simulink model "simulation"  (R2015a)
settings: Solver=ode23tb  StartTime=0.0  StopTime=0.5  RelTol=1e-3
libraries: powerlib x16
settings Model: Creator=user  LastModifiedBy=user

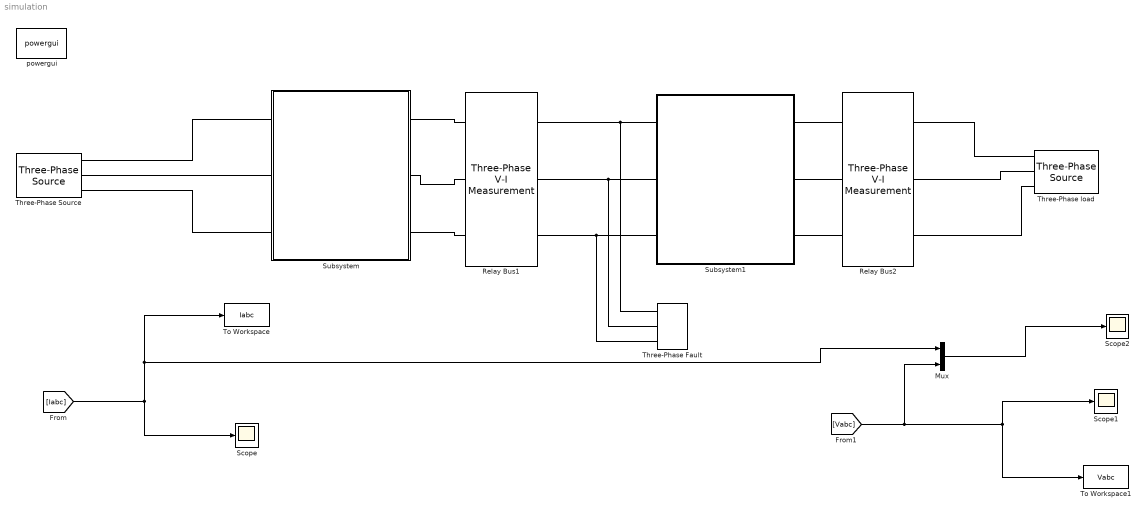
== system simulation ==
  Mux : Mux  Inputs=2
  Relay Bus1 : powerlib/Measurements/Three-Phase V-I Measurement  VoltageMeasurement=phase-to-phase  SetLabelV=on  LabelV=Vabc  Vpu=on  VpuLL=off  CurrentMeasurement=yes  SetLabelI=on  LabelI=Iabc  Ipu=on  Pbase=100e6  Vbase=500e3  OutputType=Complex  PhasorSimulation=off  PSBequivalent=0
  Relay Bus2 : powerlib/Measurements/Three-Phase V-I Measurement  VoltageMeasurement=no  SetLabelV=off  LabelV=Vabc  Vpu=on  VpuLL=off  CurrentMeasurement=no  SetLabelI=off  LabelI=Iabc  Ipu=on  Pbase=100e6  Vbase=500e3  OutputType=Complex  PhasorSimulation=off  PSBequivalent=0
  Scope : Scope
  Scope1 : Scope
  Scope2 : Scope
      settings: SaveName=ScopeData2
  Subsystem : Subsystem
  Subsystem1 : Subsystem
  Three-Phase Fault : powerlib/Elements/Three-Phase Fault  InitialStates=0  FaultA=on  FaultB=off  FaultC=off  GroundFault=on  SwitchTimes="[1/60  5/60]"  External=off  SwitchStatus=NaN  FaultResistance=0.001  GroundResistance=0.01  SnubberResistance=1e6  SnubberCapacitance=inf  Measurements=Fault voltages and currents
  Three-Phase Source : powerlib/Electrical Sources/Three-Phase Source  Voltage=500e3  PhaseAngle=0  Frequency=50  InternalConnection=Yg  SpecifyImpedance=off  Resistance=0.8929  Inductance=16.58e-3  ShortCircuitLevel=100e6  BaseVoltage=500e3  XRratio=7  BusType=swing  Pref=0  Qref=0  Qmin=-inf  Qmax=inf
  Three-Phase load : powerlib/Electrical Sources/Three-Phase Source  Voltage=500e3  PhaseAngle=-30  Frequency=50  InternalConnection=Yg  SpecifyImpedance=off  Resistance=0.8929  Inductance=16.58e-3  ShortCircuitLevel=100e6  BaseVoltage=500e3  XRratio=7  BusType=swing  Pref=0  Qref=0  Qmin=-inf  Qmax=inf
  To Workspace : ToWorkspace  VariableName=Iabc  SaveFormat=Timeseries
  To Workspace1 : ToWorkspace  VariableName=Vabc  SaveFormat=Timeseries
  powergui : powerlib/powergui  Priority=1  SimulationMode=Discrete  SolverType=Tustin/Backward Euler (TBE)  SampleTime=3e-5  frequency=60  SPID=off  DisableSnubberDevices=off  DisableRonSwitches=off  DisableVfSwitches=off  SwTol=0  DisplayEquations=off  Interpol=off  methode=off  Ts=100  FunctionMessages=off  echomessages=off  HookPort=off  EnableUseOfTLC=off  x0status=blocks  frequencyindice=50  Pbase=100e6  ErrMax=1e-4  Iterations=50  UnitsV=kV  UnitsW=MW  buscounter=0  RestoreLinks=warning  ResistiveCurrentMeasurement=off  Frange=[0:2:500]  Ylog=off  Xlog=on  ShowGrid=off  save=off  variable=ZData  structure=0  ZoomFFT=off  StartTime=0.0  cycles=1  DisplayStyle=1  fundamental=60  FreqAxis=off  MaxFrequency=1000  frequencyindicesteady=1  RmsSteady=1  display=off
  wires:
  [Iabc] -> Scope/1, Mux/1, To Workspace/1
  [Vabc] -> Mux/2, Scope1/1, To Workspace1/1
  Mux/1 -> Scope2/1
  connections:
  Relay Bus1/LConn2 -- Subsystem/RConn2
  Three-Phase Source/RConn1 -- Subsystem/LConn1
  Three-Phase Source/RConn2 -- Subsystem/LConn2
  Three-Phase Source/RConn3 -- Subsystem/LConn3
  Subsystem/RConn1 -- Relay Bus1/LConn1
  Subsystem/RConn3 -- Relay Bus1/LConn3
  Three-Phase load/RConn2 -- Relay Bus2/RConn2
  Three-Phase load/RConn3 -- Relay Bus2/RConn3
  Three-Phase load/RConn1 -- Relay Bus2/RConn1
  Subsystem1/RConn1 -- Relay Bus2/LConn1
  Subsystem1/RConn2 -- Relay Bus2/LConn2
  Subsystem1/RConn3 -- Relay Bus2/LConn3
  Relay Bus1/RConn2 -- Three-Phase Fault/LConn2 -- Subsystem1/LConn2
  Relay Bus1/RConn1 -- Three-Phase Fault/LConn1 -- Subsystem1/LConn1
  Relay Bus1/RConn3 -- Three-Phase Fault/LConn3 -- Subsystem1/LConn3

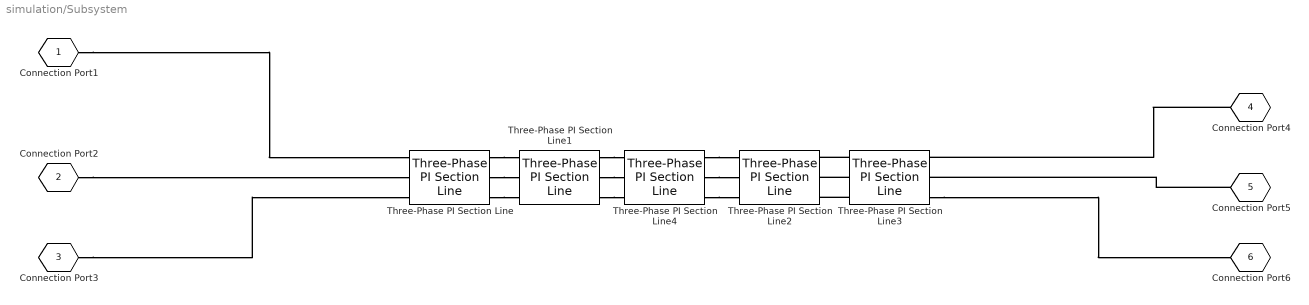
== system simulation/Subsystem ==
  Three-Phase PI Section Line{,1..4} (5 alike) : powerlib/Elements/Three-Phase PI Section Line  LConnTagsString=a|b|c  RConnTagsString=A|B|C  Frequency=50  Resistances=[ 0.01273 0.3864]  Inductances="[ 0.9337e-3  4.1264e-3]"  Capacitances=[12.74e-9 7.751e-9]  Length=30
  Connection Port1 : PMIOPort  Tag=PMCPort  Port=1  Side=Right
  Connection Port2 : PMIOPort  Tag=PMCPort  Port=2  Side=Left
  Connection Port3 : PMIOPort  Tag=PMCPort  Port=3  Side=Left
  Connection Port4 : PMIOPort  Tag=PMCPort  Port=4  Side=Right
  Connection Port5 : PMIOPort  Tag=PMCPort  Port=5  Side=Left
  Connection Port6 : PMIOPort  Tag=PMCPort  Port=6  Side=Right
  connections:
  Three-Phase PI Section Line4/RConn2 -- Three-Phase PI Section Line2/LConn2
  Three-Phase PI Section Line4/RConn3 -- Three-Phase PI Section Line2/LConn3
  Connection Port3/RConn1 -- Three-Phase PI Section Line/LConn3
  Connection Port1/RConn1 -- Three-Phase PI Section Line/LConn1
  Connection Port2/RConn1 -- Three-Phase PI Section Line/LConn2
  Three-Phase PI Section Line4/RConn1 -- Three-Phase PI Section Line2/LConn1
  Three-Phase PI Section Line/RConn3 -- Three-Phase PI Section Line1/LConn3
  Three-Phase PI Section Line/RConn1 -- Three-Phase PI Section Line1/LConn1
  Three-Phase PI Section Line3/LConn3 -- Three-Phase PI Section Line2/RConn3
  Three-Phase PI Section Line3/LConn1 -- Three-Phase PI Section Line2/RConn1
  Three-Phase PI Section Line3/LConn2 -- Three-Phase PI Section Line2/RConn2
  Three-Phase PI Section Line/RConn2 -- Three-Phase PI Section Line1/LConn2
  Three-Phase PI Section Line1/RConn3 -- Three-Phase PI Section Line4/LConn3
  Three-Phase PI Section Line1/RConn2 -- Three-Phase PI Section Line4/LConn2
  Three-Phase PI Section Line1/RConn1 -- Three-Phase PI Section Line4/LConn1
  Connection Port5/RConn1 -- Three-Phase PI Section Line3/RConn2
  Three-Phase PI Section Line3/RConn3 -- Connection Port6/RConn1
  Connection Port4/RConn1 -- Three-Phase PI Section Line3/RConn1

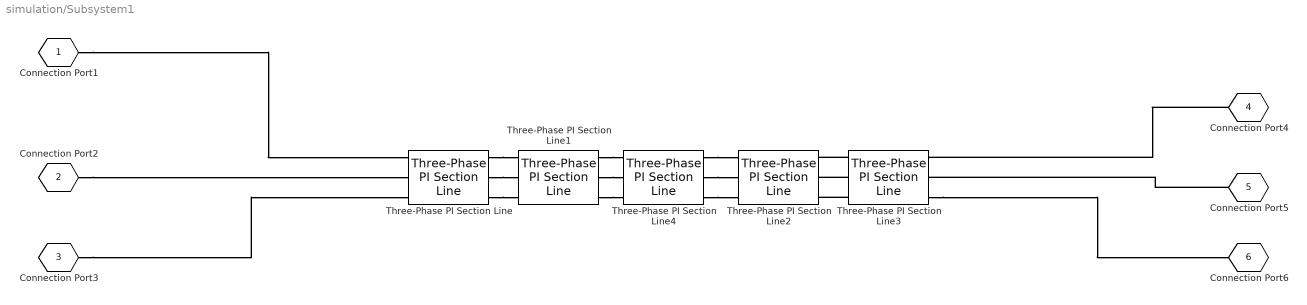
== system simulation/Subsystem1 ==
  Three-Phase PI Section Line{,1..4} (5 alike) : powerlib/Elements/Three-Phase PI Section Line  LConnTagsString=a|b|c  RConnTagsString=A|B|C  Frequency=50  Resistances=[ 0.01273 0.3864]  Inductances="[ 0.9337e-3  4.1264e-3]"  Capacitances=[12.74e-9 7.751e-9]  Length=30
  Connection Port1 : PMIOPort  Tag=PMCPort  Port=1  Side=Right
  Connection Port2 : PMIOPort  Tag=PMCPort  Port=2  Side=Left
  Connection Port3 : PMIOPort  Tag=PMCPort  Port=3  Side=Left
  Connection Port4 : PMIOPort  Tag=PMCPort  Port=4  Side=Right
  Connection Port5 : PMIOPort  Tag=PMCPort  Port=5  Side=Left
  Connection Port6 : PMIOPort  Tag=PMCPort  Port=6  Side=Right
  connections:
  Three-Phase PI Section Line4/RConn2 -- Three-Phase PI Section Line2/LConn2
  Three-Phase PI Section Line4/RConn3 -- Three-Phase PI Section Line2/LConn3
  Connection Port3/RConn1 -- Three-Phase PI Section Line/LConn3
  Connection Port1/RConn1 -- Three-Phase PI Section Line/LConn1
  Connection Port2/RConn1 -- Three-Phase PI Section Line/LConn2
  Three-Phase PI Section Line4/RConn1 -- Three-Phase PI Section Line2/LConn1
  Three-Phase PI Section Line/RConn3 -- Three-Phase PI Section Line1/LConn3
  Three-Phase PI Section Line/RConn1 -- Three-Phase PI Section Line1/LConn1
  Three-Phase PI Section Line3/LConn3 -- Three-Phase PI Section Line2/RConn3
  Three-Phase PI Section Line3/LConn1 -- Three-Phase PI Section Line2/RConn1
  Three-Phase PI Section Line3/LConn2 -- Three-Phase PI Section Line2/RConn2
  Three-Phase PI Section Line/RConn2 -- Three-Phase PI Section Line1/LConn2
  Three-Phase PI Section Line1/RConn3 -- Three-Phase PI Section Line4/LConn3
  Three-Phase PI Section Line1/RConn2 -- Three-Phase PI Section Line4/LConn2
  Three-Phase PI Section Line1/RConn1 -- Three-Phase PI Section Line4/LConn1
  Connection Port5/RConn1 -- Three-Phase PI Section Line3/RConn2
  Three-Phase PI Section Line3/RConn3 -- Connection Port6/RConn1
  Connection Port4/RConn1 -- Three-Phase PI Section Line3/RConn1
